simulink model "HW3"  (R2022b)
settings: Solver=VariableStepAuto  StartTime=0.0  StopTime=10.0  RelTol=1e-3
values from neighbouring files (symbols this model uses):
  A = 4*1e-4    (= 0.0004)    [Variables.m]    (also in vars.m)
  e = i*R    [Variables.m]
  fd_f = 10    [Variables.m]    (also in vars.m = 1)
  fd_m = 1e-4    (= 0.0001)    [Variables.m]    (also in vars.m)
  g = 5*1e-4    (= 0.0005)    [Variables.m]    (also in vars.m)
  i = sqrt(2*K_s*(x_i-x)*(x+g)^2/(N^2*mu_0*A))    [Variables.m]
  K_s = 100    [Variables.m]    (also in vars.m)
  m = 0.05    [Variables.m]    (also in vars.m)
  mu_0 = 4*pi*1e-7    (= 1.25663706144e-06)    [Variables.m]    (also in vars.m)
  N = 100    [Variables.m]    (also in vars.m)
  R = 1    [Variables.m]    (also in vars.m)
  v = 0    [Variables.m]
  x_i = 1e-2    (= 0.01)    [Variables.m]    (also in vars.m)
settings Model: VariantFading=off  Creator=qingchuanhou  LastModifiedBy=qingchuanhou

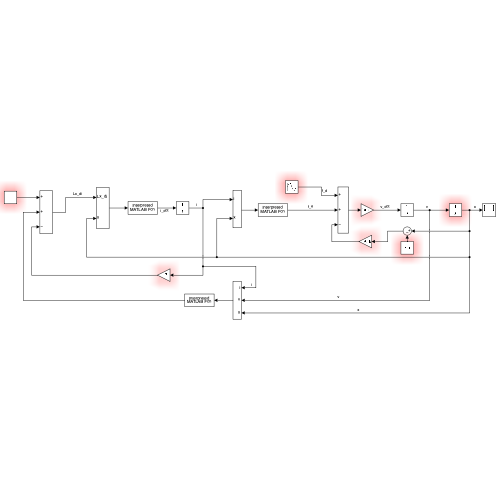
[thumbnail: Simulink's stored preview of the top-level diagram]
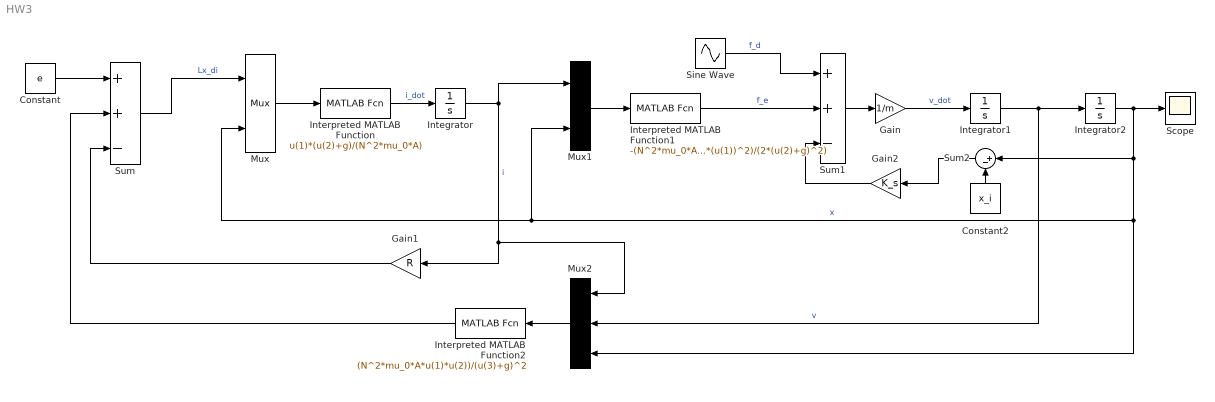
== system HW3 ==
  Constant : Constant  Value=e
  Constant2 : Constant  Value=x_i
  Gain : Gain  Gain=1/m
  Gain1 : Gain  Gain=R
  Gain2 : Gain  Gain=K_s
  Integrator : Integrator  InitialCondition=i
  Integrator1 : Integrator
  Integrator2 : Integrator  InitialCondition=v
  Interpreted MATLAB Function : MATLABFcn  MATLABFcn=u(1)*(u(2)+g)/(N^2*mu_0*A)
  Interpreted MATLAB Function1 : MATLABFcn  MATLABFcn=-(N^2*mu_0*A*(u(1))^2)/(2*(u(2)+g)^2)
  Interpreted MATLAB Function2 : MATLABFcn  MATLABFcn=(N^2*mu_0*A*u(1)*u(2))/(u(3)+g)^2
  Mux : Mux  Inputs=2
      settings: DisplayOption=signals
  Mux1 : Mux  Inputs=2
      settings: DisplayOption=signals
  Mux2 : Mux  Inputs=3
      settings: DisplayOption=signals
  Scope : Scope
  Sine Wave : Sin  Amplitude=fd_m  Frequency=fd_f  SampleTime=0
  Sum : Sum  Inputs=++-
  Sum1 : Sum  Inputs=++-
  Sum2 : Sum  Inputs=|+-
  wires:
  Interpreted MATLAB Function/1 -> Integrator/1  "i_dot"
  Integrator/1 -> Mux1/1, Mux2/1, Gain1/1  "i"
  Interpreted MATLAB Function1/1 -> Sum1/2  "f_e"
  Gain1/1 -> Sum/3
  Integrator2/1 -> Scope/1, Mux2/3, Mux/2, Mux1/2, Sum2/1  "x"
  Integrator1/1 -> Mux2/2, Integrator2/1  "v"
  Gain/1 -> Integrator1/1  "v_dot"
  Sum1/1 -> Gain/1
  Sine Wave/1 -> Sum1/1  "f_d"
  Constant2/1 -> Sum2/2
  Sum2/1 -> Gain2/1
  Gain2/1 -> Sum1/3
  Mux2/1 -> Interpreted MATLAB Function2/1
  Constant/1 -> Sum/1
  Sum/1 -> Mux/1  "Lx_di"
  Mux/1 -> Interpreted MATLAB Function/1
  Mux1/1 -> Interpreted MATLAB Function1/1
  Interpreted MATLAB Function2/1 -> Sum/2
